simulink model "optotrak_single_pendulum_and_VR_v2"  (R2019b)
settings: Solver=ode3  StartTime=0.0  StopTime=inf  FixedStep=0.01  RelTol=1e-3  EnableMultiTasking=on
libraries: mblibv1 x3, xpcrtudplib x2, xpcutilitieslib x2, vrlib x2, slrtlib x1
(part 2 of 2)

== matlab function optotrak_single_pendulum_and_VR_v2/OPTOTRAK Certus/Embedded MATLAB Function19 ==
  data: M_rot output; M input
function M_rot=rot_v_gl(M)
% Roman Kamnik, avgust 2010


%  ORotacija markerjev v globalni ks
% kot je pri veslanju



%  H matrika pripeta na segment - lokalni ks
% osi koordinatenga sistema

R = roty(pi/2)*rotx(pi/2);

 
M_rot = R * M(:) + [0.010125 ; 0.11977 ; 0.0];
 

%M_rot = M(:);
 
return;



%%%%%%%%%%%%%%%%%%%%%%%%%%%%%%%%%%%%%%%%%%%%%%%%%%%%%%%%%%%%%%%%%%%%%%%%

function u = unit(v)
	%u = v / norm(v,'fro');
    u = v / norm(v,2);
return    

% %%%%%%%%%%%%%%%%%%%%%%%%%%%%%%%%%%%%%%%%%%%%%%%%%%%%%%%%%%%%%%%%%%%%%%%%%
function r = rotz(t)
	ct = cos(t);
	st = sin(t);
	r =    [ct	-st	0	
		st	ct	0	
		0	0	1	];
return
% %%%%%%%%%%%%%%%%%%%%%%%%%%%%%%%%%%%%%%%%%%%%%%%%%%%%%%%%%%%%%%%%%%%%%%%%%

function r = rotx(t)
	ct = cos(t);
	st = sin(t);
	r =[1	0	0;...	
		0	ct	-st;...	
		0	st	ct	];
return    
  % %%%%%%%%%%%%%%%%%%%%%%%%%%%%%%%%%%%%%%%%%%%%%%%%%%%%%%%%%%%%%%%%%%%%%%%%%
  
function r = roty(t)
	ct = cos(t);
	st = sin(t);
	r =    [ct	0	st	
            0	1	0	
            -st	0	ct	];
return
% %%%%%%%%%%%%%%%%%%%%%%%%%%%%%%%%%%%%%%%%%%%%%%%%%%%%%%%%%%%%%%%%%%%%%%%%%
